simulink model "ex02_model"  (R2023a)
settings: Solver=FixedStepDiscrete  StartTime=0.0  StopTime=100*Ts  RelTol=1e-3
values from neighbouring files (symbols this model uses):
  Fc = 1e3    (= 1000)    [ex01_config.m]    (also in ex02_config.m)
  Ts = 1/Fs    (= 6.25e-05)    [ex01_config.m]    (also in ex02_config.m)
libraries: dspsrcs4 x1, dspsigops x1
settings Model: Creator=daniele  LastModifiedBy=daniele
settings SolverCC: AlgebraicLoopSolver=TrustRegion
settings DataIOCC: ReturnWorkspaceOutputs=off
settings DebuggingCC: UnconnectedInputMsg=warning  UnconnectedOutputMsg=warning  UnconnectedLineMsg=warning  ArithmeticOperatorsInVariantConditions=warning
settings ModelReferenceCC: EnableRefExpFcnMdlSchedulingChecks=on
settings SFSimCC: CustomCodeUndefinedFunction=UseInterfaceOnly

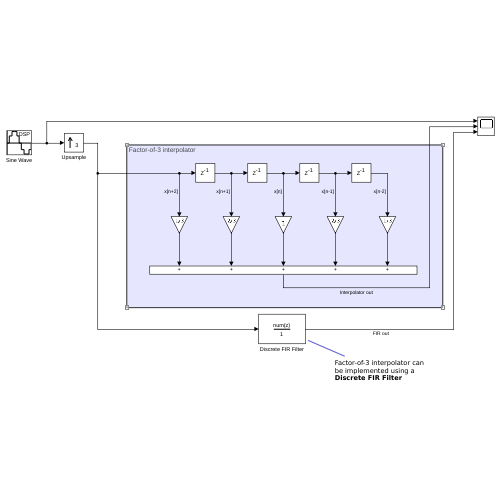
[thumbnail: Simulink's stored preview of the top-level diagram]
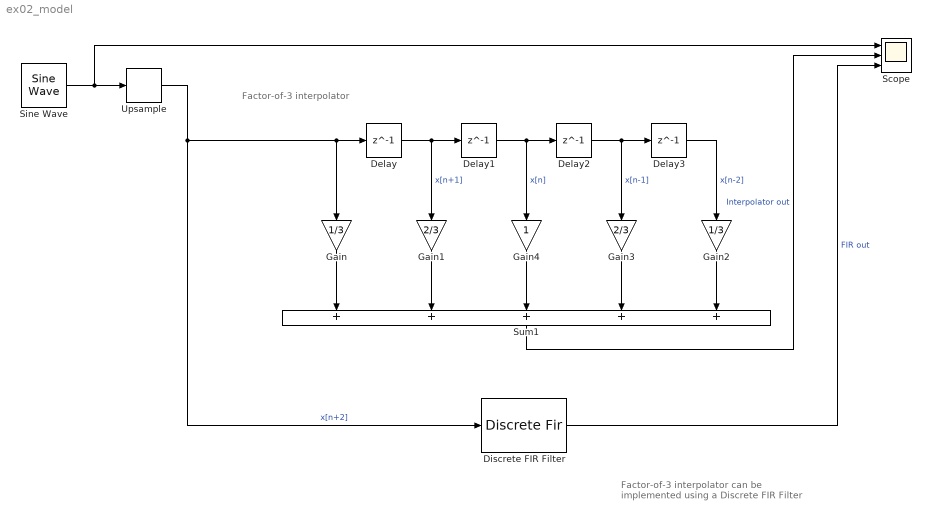
== system ex02_model ==
  note: Factor-of-3 interpolator can be implemented using a Discrete FIR Filter
  note: Factor-of-3 interpolator
  Delay{,1..3} (4 alike) : Delay  DelayLength=1
  Discrete FIR Filter : DiscreteFir  Coefficients=[1/3 2/3 1 2/3 1/3]
  Gain : Gain  Gain=1/3
  Gain1 : Gain  Gain=2/3
  Gain2 : Gain  Gain=1/3
  Gain3 : Gain  Gain=2/3
  Gain4 : Gain
  Scope : Scope  NumInputPorts=3
  Sine Wave : dspsrcs4/Sine Wave  Amplitude=1  Frequency=Fc  Phase=pi/2  SampleMode=Discrete  OutComplex=Real  CompMethod=Trigonometric fcn  TableSize=Speed  SampleTime=Ts  SamplesPerFrame=1  ResetState=Restart at time zero  OutputFrames=off  dataType=double  wordLen=16  udDataType=sfix(16)  fracBitsMode=Best precision  numFracBits=15  OutDataTypeStr=double  LastOutDataTypeStr=double
  Sum1 : Sum  Inputs=+++++
  Upsample : dspsigops/Upsample  FactorSource=Dialog parameter  N=3  Nmax=16  phase=0  RateOptions=Allow multirate processing  ic=0  mode=Unused parameter value
      settings: LibrarySourceBlock=dsphdlsupportsigops/Upsample
  wires:
  Delay/1 -> Gain1/1, Delay1/1  "x[n+1]"
  Delay1/1 -> Delay2/1, Gain4/1  "x[n]"
  Gain1/1 -> Sum1/2
  Gain/1 -> Sum1/1
  Gain3/1 -> Sum1/4
  Delay3/1 -> Gain2/1  "x[n-2]"
  Sine Wave/1 -> Scope/1, Upsample/1
  Delay2/1 -> Delay3/1, Gain3/1  "x[n-1]"
  Upsample/1 -> Gain/1, Delay/1, Discrete FIR Filter/1  "x[n+2]"
  Gain2/1 -> Sum1/5
  Sum1/1 -> Scope/2  "Interpolator out"
  Discrete FIR Filter/1 -> Scope/3  "FIR out"
  Gain4/1 -> Sum1/3
